simulink model "px4_rate_control"  (R2022b)
settings: Solver=FixedStepAuto  StartTime=0.0  StopTime=inf  RelTol=1e-3
values from neighbouring files (symbols this model uses):
  lb = 0    [Initialization_Simulink.m]
  lbu = -inf(nu,1)    [InitData.m]    (also in Initialization_Simulink.m = repmat(lbu,1,N))
  lbx = 0    [Initialization_Simulink.m]
  para = repmat(para0,1,N+1)    [InitData.m]    (also in Initialization_Simulink.m)
  Ts = settings.Ts_st    [Initialization_Simulink.m]    (also in Simulation.m)
  ub = 0    [Initialization_Simulink.m]
  ubu = inf(nu,1)    [InitData.m]    (also in Initialization_Simulink.m = repmat(ubu,1,N))
  ubx = 0    [Initialization_Simulink.m]
  W = repmat([Qp Qrpy Qq Qv Qu]',1,N)    [Initialization_Simulink.m]
  WN = [Qp Qrpy Qq Qv]'    [Initialization_Simulink.m]
  z0 = 0    [Initialization_Simulink.m]
undefined symbols (not defined in the file or in its folder): body_rate, opt, pitch, roll, settings, thrust_body, timestamp, yaw
libraries: ros2lib x6, aerolibutil x6, robotcorelib x1
settings Model: Creator=beniamino  LastModifiedBy=beniamino
settings OptimizationCC: EnhancedBackFolding=on  PassReuseOutputArgsAs=Individual arguments  ZeroExternalMemoryAtStartup=off  ZeroInternalMemoryAtStartup=off  MaxStackSize=64  OptimizeBlockOrder=speed  DifferentSizesBufferReuse=on  OptimizationCustomize=off  EfficientTunableParamExpr=on
settings DebuggingCC: ParameterTunabilityLossMsg=error
settings HardwareCC: ProdBitPerLong=64  ProdHWDeviceType=Intel->x86-64 (Linux 64)
settings SFSimCC: MATLABDynamicMemAlloc=off
settings RTWCC: Description=Embedded Coder  SystemTargetFile=ert.tlc  HardwareBoard=Robot Operating System 2 (ROS 2)  TLCOptions="-aInlineSetEventsForThisBaseRateFcn=TLC_FALSE -aSuppressMultiTaskScheduler=TLC_FALSE  -aRateBasedStepFcn=0"  TemplateMakefile=ert_default_tmf  Toolchain=Colcon Tools  TargetLang=C++
settings CodeAppCC: ForceParamTrailComments=on  IgnoreCustomStorageClasses=off  OperatorAnnotations=on  SimulinkDataObjDesc=on  SFDataObjDesc=on  InsertBlockDesc=on
settings ERTTargetCC: CodeInterfacePackaging=C++ class  RootIOFormat=Structure reference

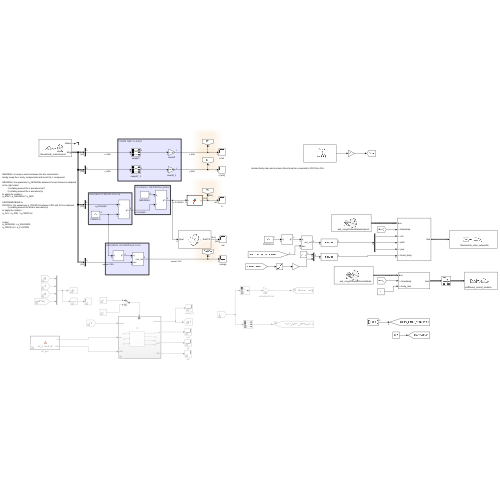
[thumbnail: Simulink's stored preview of the top-level diagram]
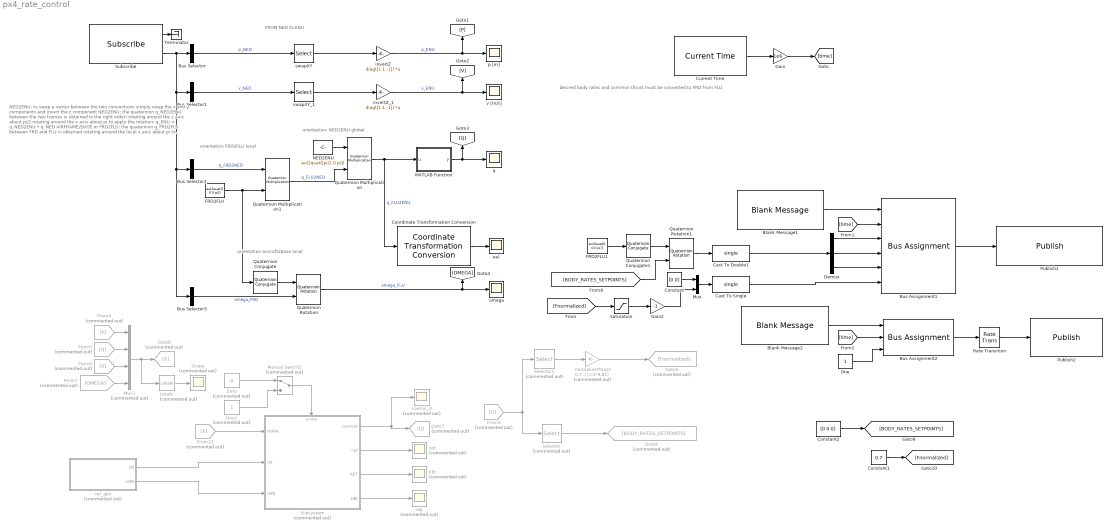
== system px4_rate_control ==
  note: desired body rates and common thrust must be converted to FRD from FLU
  note: orientation FRD2FLU local
  note: orientation: NED2ENU global
  note: FROM NED to ENU
  note: orientation aircraft2base local
  note: NED2ENU: to swap a vector between the two conventions
      | simply swap the x and y components and invert the z component
      |
      | NED2ENU: the quaternion q_NED2ENU between the two frames is obtained
      | in the right order!
      | rotating around the z axis about pi/2
      | rotating around the x axis about pi
      | to apply the rotation:
      | q_ENU = q_NED2ENU * q_NED
      |
      | AIRFRAME2BASE or
      | FRD2FLU: the quaternion q_FRD2FLU between FRD and FLU is obtained
      | rotating around the local x axis about pi
      | to apply the rotation
      | q_FLU = q_FRD * q_FRD2FLU
      |
      | notice!
      | q_NED2ENU = q_ENU2NED
      | q_FRD2FLU = q_FLU2FRD
  Blank Message1 : ros2lib/Blank Message  messageClass=Message  entityType=px4_msgs/VehicleRatesSetpoint  messageType=px4_msgs/VehicleRatesSetpoint  SampleTime=inf
      settings: LibrarySourceBlock=roslib/ROS 2/Blank Message
  Blank Message2 : ros2lib/Blank Message  messageClass=Message  entityType=px4_msgs/OffboardControlMode  messageType=px4_msgs/OffboardControlMode  SampleTime=inf
      settings: LibrarySourceBlock=roslib/ROS 2/Blank Message
  Bus Assignment1 : BusAssignment  AssignedSignals=timestamp,roll,pitch,yaw,thrust_body
  Bus Assignment2 : BusAssignment  AssignedSignals=timestamp,body_rate
  Bus Selector : BusSelector  OutputSignals=position  OutputAsBus=on
  Bus Selector1 : BusSelector  OutputSignals=velocity  OutputAsBus=on
  Bus Selector2 : BusSelector  OutputSignals=q  OutputAsBus=on
  Bus Selector3 : BusSelector  OutputSignals=angular_velocity  OutputAsBus=on
  Cast To Double1 : DataTypeConversion  OutDataTypeStr=single  SaturateOnIntegerOverflow=off  RndMeth=Floor
  Cast To Single : DataTypeConversion  OutDataTypeStr=single  SaturateOnIntegerOverflow=off  RndMeth=Floor
  Constant : Constant  Value=[0 0]
  Constant1 : Constant  Value=0.7
  Constant2 : Constant  Value=[0 0 0]
  Coordinate Transformation Conversion : robotcorelib/Coordinate Transformation Conversion  InputRepresentation=Quaternion  InputEulerSequence=ZYX  ShowTrVecInputPort=on  OutputRepresentation=Euler Angles  OutputEulerSequence=ZYX  ShowTrVecOutputPort=on  SimulateUsing=Code generation
      settings: LibrarySourceBlock=roslib/Utilities/Coordinate Transformation Conversion
  Current Time : ros2lib/Current Time  OutputFormat=double  SampleTime=0.01  ModelName=px4_rate_control
      settings: LibrarySourceBlock=roslib/ROS 2/Current Time
  Demux : Demux  Outputs=3
  FRD2FLU : Constant  Value=eul2quat([ 0 0 pi])  OutDataTypeStr=single
  FRD2FLU1 : Constant  Value=eul2quat([ 0 0 pi])
  From13 : From  Commented=on  GotoTag=X
  From3 : From  Commented=on  GotoTag=U
  From4 : From  Commented=on  GotoTag=P
  From5 : From  Commented=on  GotoTag=Q
  From6 : From  Commented=on  GotoTag=V
  From7 : From  Commented=on  GotoTag=OMEGA
  Gain : Gain  Gain=1e6
  Gain2 : Gain  Gain=-1
  Goto5 : Goto  Commented=on  GotoTag=Fnormalized
  Goto6 : Goto  Commented=on  GotoTag=BODY_RATES_SETPOINTS
  Goto7 : Goto  Commented=on  GotoTag=U
  Goto8 : Goto  Commented=on  GotoTag=X
  IsNaN : RelationalOperator  Commented=on  Operator=isNaN  OutDataTypeStr=boolean  RndMeth=Simplest  InputSameDT=off
  MATLAB Function : MATLAB Function  TreatAsAtomicUnit=on
  Manual Switch1 : ManualSwitch  Commented=on
  Mux : Mux  Inputs=2
  Mux1 : Mux  Commented=on
  NED2ENU : Constant  Value=eul2quat([pi/2 0 pi])  OutDataTypeStr=single
  One : Constant  OutDataTypeStr=boolean
  One1 : Constant  Commented=on  OutDataTypeStr=Inherit: Inherit via back propagation
  Publish1 : ros2lib/Publish  topicSource=Select from ROS network  topic=/fmu/vehicle_rates_setpoint/in  messageType=px4_msgs/VehicleRatesSetpoint  QOSHistory=Keep last  QOSDepth=1  QOSReliability=Best effort  QOSDurability=Volatile
      settings: LibrarySourceBlock=roslib/ROS 2/Publish
  Publish2 : ros2lib/Publish  topicSource=Select from ROS network  topic=/fmu/offboard_control_mode/in  messageType=px4_msgs/OffboardControlMode  QOSHistory=Keep last  QOSDepth=1  QOSReliability=Best effort  QOSDurability=Volatile
      settings: LibrarySourceBlock=roslib/ROS 2/Publish
  Quaternion Conjugate : aerolibutil/Quaternion Conjugate
  Quaternion Conjugate1 : aerolibutil/Quaternion Conjugate
  Quaternion Multiplication : aerolibutil/Quaternion Multiplication
  Quaternion Multiplication1 : aerolibutil/Quaternion Multiplication
  Quaternion Rotation : aerolibutil/Quaternion Rotation
  Quaternion Rotation1 : aerolibutil/Quaternion Rotation
  Rate Transition : RateTransition  OutPortSampleTime=0.1
  Saturation : Saturate  UpperLimit=1  LowerLimit=0
  Scope : Scope  Commented=on
  Selector : Selector  Commented=on  InputPortWidth=4  IndexOptions=Index vector (dialog)  Indices=2:4  OutputSizes=1
  Selector1 : Selector  Commented=on  InputPortWidth=4  IndexOptions=Index vector (dialog)  Indices=1  OutputSizes=1
  Subscribe : ros2lib/Subscribe  topicSource=Select from ROS network  topic=/fmu/vehicle_odometry/out  messageType=px4_msgs/VehicleOdometry  sampleTime=0.01  QOSHistory=Keep last  QOSDepth=1  QOSReliability=Reliable  QOSDurability=Volatile
      settings: LibrarySourceBlock=roslib/ROS 2/Subscribe
  Subsystem : Subsystem  Commented=on
  Terminator : Terminator
  Zero : Constant  Commented=on  Value=0  OutDataTypeStr=Inherit: Inherit via back propagation
  control_0 : Scope  Commented=on
  cpt : Scope  Commented=on
  eul : Scope
  invertZ : Gain  Gain=diag([1 1 -1])  Multiplication=Matrix(K*u) (u vector)
  invertZ_1 : Gain  Gain=diag([1 1 -1])  Multiplication=Matrix(K*u) (u vector)
  kkt : Scope  Commented=on
  normalizeThrust : Gain  Commented=on  Gain=0.7 ./ (1.5*9.81)
  obj : Scope  Commented=on
  omega : Scope
  p [m] : Scope
  q : Scope
  ref_gen : MATLAB Function  Commented=on  TreatAsAtomicUnit=on
  swapXY : Selector  InputPortWidth=3  IndexOptions=Index vector (dialog)  Indices=[2 1 3]  OutputSizes=1
  swapXY_1 : Selector  InputPortWidth=3  IndexOptions=Index vector (dialog)  Indices=[2 1 3]  OutputSizes=1
  v [m/s] : Scope
  wires:
  Subscribe/2 -> Bus Selector1/1, Bus Selector3/1, Bus Selector2/1, Bus Selector/1
  Bus Selector/1 -> swapXY/1  "p_NED"
  invertZ/1 -> p [m]/1, [P]  "p_ENU"
  swapXY/1 -> invertZ/1
  Bus Selector1/1 -> swapXY_1/1  "v_NED"
  swapXY_1/1 -> invertZ_1/1
  invertZ_1/1 -> [V], v [m/s]/1  "v_ENU"
  Bus Selector2/1 -> Quaternion Multiplication1/1  "q_FRD2NED"
  Quaternion Multiplication/1 -> Coordinate Transformation Conversion/1, MATLAB Function/1(u)  "q_FLU2ENU"
  NED2ENU/1 -> Quaternion Multiplication/1
  Subscribe/1 -> Terminator/1
  Quaternion Multiplication1/1 -> Quaternion Multiplication/2  "q_FLU2NED"
  FRD2FLU/1 -> Quaternion Conjugate/1, Quaternion Multiplication1/2
  Coordinate Transformation Conversion/1 -> eul/1
  Bus Selector3/1 -> Quaternion Rotation/2  "omega_FRD"
  Quaternion Conjugate/1 -> Quaternion Rotation/1
  Quaternion Rotation/1 -> [OMEGA], omega/1  "omega_FLU"
  Blank Message1/1 -> Bus Assignment1/1
  [time] -> Bus Assignment1/2
  [BODY_RATES_SETPOINTS] -> Quaternion Rotation1/2
  Bus Assignment1/1 -> Publish1/1
  Blank Message2/1 -> Bus Assignment2/1
  [time] -> Bus Assignment2/2
  One/1 -> Bus Assignment2/3
  Bus Assignment2/1 -> Rate Transition/1
  Rate Transition/1 -> Publish2/1
  Quaternion Conjugate1/1 -> Quaternion Rotation1/1
  FRD2FLU1/1 -> Quaternion Conjugate1/1
  Cast To Double1/1 -> Demux/1
  Quaternion Rotation1/1 -> Cast To Double1/1
  Selector1/1 -> normalizeThrust/1
  Selector/1 -> Goto6/1
  Demux/1 -> Bus Assignment1/3
  Demux/2 -> Bus Assignment1/4
  Demux/3 -> Bus Assignment1/5
  Cast To Single/1 -> Bus Assignment1/6
  Mux/1 -> Cast To Single/1
  Constant/1 -> Mux/1
  Gain2/1 -> Mux/2
  Saturation/1 -> Gain2/1
  [Fnormalized] -> Saturation/1
  normalizeThrust/1 -> Goto5/1
  One1/1 -> Manual Switch1/2
  Zero/1 -> Manual Switch1/1
  Manual Switch1/1 -> Subsystem/Enable
  Subsystem/4(OBJ) -> obj/1
  Subsystem/3(KKT) -> kkt/1
  Subsystem/2(cpt) -> cpt/1
  ref_gen/2(refN) -> Subsystem/3(refN)
  ref_gen/1(ref) -> Subsystem/2(ref)
  From13/1 -> Subsystem/1(states)
  Subsystem/1(controls) -> control_0/1, Goto7/1
  From3/1 -> Selector/1, Selector1/1
  Mux1/1 -> IsNaN/1, Goto8/1
  From4/1 -> Mux1/1
  From5/1 -> Mux1/2
  From6/1 -> Mux1/3
  From7/1 -> Mux1/4
  IsNaN/1 -> Scope/1
  MATLAB Function/1(y) -> [Q], q/1
  Constant1/1 -> [Fnormalized]
  Constant2/1 -> [BODY_RATES_SETPOINTS]
  Current Time/1 -> Gain/1
  Gain/1 -> [time]

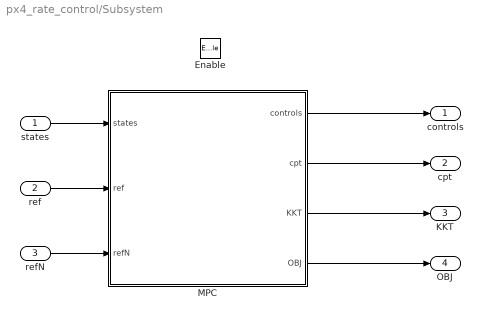
== system px4_rate_control/Subsystem ==
  states : Inport
  ref : Inport  Port=2
  refN : Inport  Port=3
  Enable : EnablePort
  MPC : MATLAB Function  TreatAsAtomicUnit=on  SystemSampleTime=Ts
  controls : Outport  OutputWhenDisabled=reset  InitialOutput=[0 0 0 0]
  cpt : Outport  Port=2
  KKT : Outport  Port=3
  OBJ : Outport  Port=4
  wires:
  states/1 -> MPC/1(states)
  ref/1 -> MPC/2(ref)
  refN/1 -> MPC/3(refN)
  MPC/1(controls) -> controls/1
  MPC/4(OBJ) -> OBJ/1
  MPC/3(KKT) -> KKT/1
  MPC/2(cpt) -> cpt/1

== matlab function px4_rate_control/ref_gen ==
  data: ref output; settings parameter; refN output
function [ref,refN] = Ref_Generator(settings)

p_ref = [2 0 2];
rpy_ref = [0 0 0];
q_ref = [1 0 0 0];
v_ref = [0 0 0];
u_ref = [14.7 0 0 0];
t_ref = [p_ref rpy_ref q_ref v_ref u_ref];
t_refN = t_ref(1:settings.nyN);

ref = repmat(t_ref',1,settings.N);
refN = t_refN';

%ref=zeros(settings.ny,settings.N);
%refN=zeros(settings.nyN,1);

%     ref = repmat([1.4, 0, 0]',1,settings.N);
%     refN = 1.4;

== matlab function px4_rate_control/MATLAB Function ==
  data: u input; y output
function y = fcn(u)
    if u(1)<0
        y=-u;
    else
        y=u;
    end

== matlab function px4_rate_control/Subsystem/MPC ==
  settings: updateMethod=DISCRETE  sampleTime=0.01
  data: states input size=nx; settings parameter; opt parameter; lb parameter; ub parameter; lbx parameter; ubx parameter; lbu parameter; ubu parameter; W parameter; WN parameter; para parameter; ref input size=[ny N]; refN input size=nyN; z0 parameter; controls output size=nu; cpt output size=1; KKT output; OBJ output
function [controls, cpt, KKT, OBJ] = NMPC_BLOCK(states, settings, opt, lb, ub, lbx, ubx, lbu, ubu, W, WN, para, ref, refN, z0)

%% everything should has a fixed size
coder.extrinsic('mpc_nmpcsolver_simulink');  
coder.extrinsic('InitData');  
coder.extrinsic('InitMemory');  
coder.extrinsic('evalin');
coder.extrinsic('assignin');

%%

persistent x u z lambda mu mu_x mu_u;
persistent input mem;

if isempty(input)  
    
    nx = settings.nx;        % No. of differential states
    nu = settings.nu;        % No. of controls
    nz = settings.nz;        % No. of algebraic states
    ny = settings.ny;        % No. of outputs (references)    
    nyN= settings.nyN;       % No. of outputs at terminal stage 
    np = settings.np;        % No. of parameters (on-line data)
    nc = settings.nc;        % No. of constraints
    ncN = settings.ncN;      % No. of constraints at terminal stage
    nbu = settings.nbu;      % No. of control bounds
    nbx = settings.nbx;      % No. of state bounds
    nbu_idx = settings.nbu_idx; % Index of control bounds
    nbx_idx = settings.nbx_idx; % Index of state bounds
    N = settings.N;
    N2 = settings.N2;
    r = settings.r;
        
    input.x0=states;
    
    x=repmat(states,1,N+1);
    input.x=x;
    
    u=zeros(nu,N);
    input.u=u;
    
    z=repmat(z0,1,N);
    input.z=z;
    
    lambda = zeros(nx,N+1);
    input.lambda= lambda;
    
    if N*nc+ncN > 0
        mu = zeros(N*nc+ncN,1);
    else
        mu = 0;
    end
    input.mu= mu;
    
    mu_u = zeros(N*nu,1);
    input.mu_u= mu_u;
    
    if N*nbx > 0
        mu_x = zeros(N*nbx,1);
    else
        mu_x = 0;
    end
    input.mu_x = mu_x;
    
    input.W=W;
    input.WN=WN;
    input.od = para;
    
    input.lb = lb;
    input.ub = ub;
    input.lbx = lbx;
    input.ubx = ubx;
    input.lbu = lbu;
    input.ubu = ubu;
      
    input.y = ref;
    input.yN = refN;
    
    mem = InitMemory(settings, opt, input);
        
else

    input.x=x; 
    input.u=u;
    input.z=z;
    input.lambda=lambda;   
    input.mu=mu;
    input.mu_x=mu_x;
    input.mu_u=mu_u;
    
end

%%
cpt = 0;
KKT = 0;
OBJ = 0;
input.x0 = states;
[input,mem,cpt,KKT,OBJ] = mpc_nmpcsolver_simulink(input, settings, mem, opt);
controls = input.u(:,1);

%% shifting
switch opt.shifting
    case 'yes'
        x=[input.x(:,2:end),input.x(:,end)];  
        u=[input.u(:,2:end),input.u(:,end)]; 
        z=[input.z(:,2:end),input.z(:,end)]; 
        lambda=[input.lambda(:,2:end),input.lambda(:,end)];
        if (settings.N*settings.nc+settings.ncN) >0
            mu(1:end-settings.ncN+1)=input.mu(settings.nc+1:settings.N*settings.nc+settings.ncN,1);
            mu(settings.N*settings.nc+1:end)=input.mu(settings.N*settings.nc+settings.ncN-settings.nc+1:settings.N*settings.nc+settings.ncN,1);
        else
            mu=0;
        end
        mu_x=[input.mu_x(2:end,1);input.mu_x(end,1)];
        mu_u=[input.mu_u(2:end,1);input.mu_u(end,1)];
   case 'no'
        x=input.x;
        u=input.u;
        z=input.z;
        lambda=input.lambda;
        mu=input.mu;
        mu_x=input.mu_x;
        mu_u=input.mu_u;
end

return
